simulink model "sst_three_phase_dab_three_levels_inv"  (R2025b)
settings: Solver=ode23tb  StartTime=0.0  StopTime=simlength  FixedStep=tc  MaxStep=tc
values from neighbouring files (symbols this model uses):
  Adrso = eye(2) + Arso*ts_inv    [init_model.m]
  Aresd_max = eye(2) + Ares_max*ts_afe    [init_model.m]
  Aresd_min = eye(2) + Ares_min*ts_afe    [init_model.m]
  Aresd_nom = eye(2) + Ares_nom*ts_afe    [init_model.m]
  Bresd = Bres*ts_afe    [init_model.m]
  CFi_dc2 = 900e-6*4    (= 0.0036)    [init_model.m]
  Cresd = Cres    [init_model.m]
  Crso = [1 0]    [init_model.m]
  delta = 0.025    [init_model.m]
  freq = 50    [init_model.m]
  Iac_FS = I_phase_normalization_factor    [init_model.m]
  Idc_FS = max(Idab1_dc_nom,Idab2_dc_nom) * margin_factor    [init_model.m]
  iph_grid_pu_ref = 3.75    [init_model.m]
  ki_afe = 18    [init_model.m]
  ki_pll = 3140    [init_model.m]
  ki_rpi = 18    [init_model.m]
  kp_afe = 0.25    [init_model.m]
  kp_pll = 314    [init_model.m]
  kp_rpi = 0.25    [init_model.m]
  Ldrso = acker(Adrso',Crso',polesdrso)'    [init_model.m]
  LFu1_AFE = 0.33e-3    (= 0.00033)    [init_model.m]
  n_modules = 2    [init_model.m]
  RLFu1_AFE = 157*0.05*LFu1_AFE    (= 0.0025905)    [init_model.m]
  tc = ts_dab/1000*24    (= 1e-06)    [init_model.m]
  ts_afe = 1/fPWM_AFE    (= 0.00025)    [init_model.m]
  ts_inv = 1/fPWM_INV    (= 0.00025)    [init_model.m]
  Vac_FS = V_phase_normalization_factor    [init_model.m]
  Vdab2_dc_nom = 1500    [init_model.m]
  Vdc_FS = max(Vdab1_dc_nom,Vdab2_dc_nom) * margin_factor    [init_model.m]
undefined symbols (not defined in the file or in its folder): omega_grid_nom, V_phase_normalization_factor
libraries: fl_lib x80, nesl_utility x55, discrete_time_low_pass_filter x6, single_phase_transformer x6, pi_ctrl x4, three_phase_inverter_ideal_switch_based_model x4, three_phase_inverter_mosfet_based_with_thermal_model x4, single_phase_transformer_lib x3, three_phase_dab_modulator x2, dclink_for_three_levels x2, single_phase_three_levels_PWM_modulator x2, dq_vector_pi x2
(part 3 of 5)

== system sst_three_phase_dab_three_levels_inv/inverter_modB/single phase inverter control1/acquisition_and_scaling_current ==
  in : Inport
  1/Ti5 : Gain  Gain=1/Iac_FS  SaturateOnIntegerOverflow=on  OutDataTypeStr=Inherit: Same as input  ParamDataTypeStr=Inherit: Same as input
  out : Outport
  wires:
  in/1 -> 1/Ti5/1
  1/Ti5/1 -> out/1

== system sst_three_phase_dab_three_levels_inv/inverter_modB/single phase inverter control1/acquisition_and_scaling_dc_voltage ==
  in : Inport
  1/Ti3 : Gain  Gain=1/Vdc_FS  SaturateOnIntegerOverflow=on  OutDataTypeStr=Inherit: Same as input  ParamDataTypeStr=Inherit: Same as input
  out : Outport
  wires:
  in/1 -> 1/Ti3/1
  1/Ti3/1 -> out/1

== system sst_three_phase_dab_three_levels_inv/inverter_modB/single phase inverter control1/acquisition_and_scaling_voltage ==
  in : Inport
  1/Ti5 : Gain  Gain=1/Vac_FS  SaturateOnIntegerOverflow=on  OutDataTypeStr=Inherit: Same as input  ParamDataTypeStr=Inherit: Same as input
  out : Outport
  wires:
  in/1 -> 1/Ti5/1
  1/Ti5/1 -> out/1

== system sst_three_phase_dab_three_levels_inv/inverter_modB/single phase inverter control1/acquisition_and_scaling_voltage1 ==
  in : Inport
  1/Ti1 : Gain  Gain=1/Vac_FS  SaturateOnIntegerOverflow=on  OutDataTypeStr=Inherit: Same as input  ParamDataTypeStr=Inherit: Same as input
  1/Ti2 : Gain  Gain=1/n_modules  SaturateOnIntegerOverflow=on  OutDataTypeStr=Inherit: Same as input  ParamDataTypeStr=Inherit: Same as input
  out : Outport
  wires:
  in/1 -> 1/Ti2/1
  1/Ti1/1 -> out/1
  1/Ti2/1 -> 1/Ti1/1

== system sst_three_phase_dab_three_levels_inv/inverter_modB/single phase inverter control1/inverter_current_output_pu_reference ==
  Gain : Gain
  Rate Limiter : RateLimiter  RisingSlewLimit=50  FallingSlewLimit=-50  SampleTimeMode=inherited
  Sum : Sum  Inputs=|++
  i_out_inverter_reference_step1 : Step  Time=0.05  After=iph_grid_pu_ref  SampleTime=0
  i_out_inverter_reference_step2 : Step  Commented=on  Time=0.25  After=-iph_grid_pu_ref  SampleTime=0
  inverter_current_output_pu_reference : Outport
  wires:
  Rate Limiter/1 -> Gain/1
  Sum/1 -> Rate Limiter/1
  i_out_inverter_reference_step1/1 -> Sum/1
  i_out_inverter_reference_step2/1 -> Sum/2
  Gain/1 -> inverter_current_output_pu_reference/1

== system sst_three_phase_dab_three_levels_inv/inverter_modB/single phase inverter control1/pwm modulator ==
  vout : Inport
  Constant : Constant  Value=0
  single_phase_three_levels_PWM_generator_with_global_TRGO : single_phase_three_levels_PWM_modulator/single_phase_three_levels_PWM_generator_with_global_TRGO  f=fPWM_INV  m_up=1  m_low=-1  dead_time=dead_time_INV  pos_cmd_gate=15  neg_cmd_gate=-10  polarity=1  tc=tc  double_sampling=1
  gate_cmds : Outport
  tag scope: TRGO_INV_2=global
  wires:
  vout/1 -> single_phase_three_levels_PWM_generator_with_global_TRGO/3
  Constant/1 -> single_phase_three_levels_PWM_generator_with_global_TRGO/2
  single_phase_three_levels_PWM_generator_with_global_TRGO/2 -> gate_cmds/1
  single_phase_three_levels_PWM_generator_with_global_TRGO/1 -> [TRGO_INV_2]
  [time_afe_module_2] -> single_phase_three_levels_PWM_generator_with_global_TRGO/1

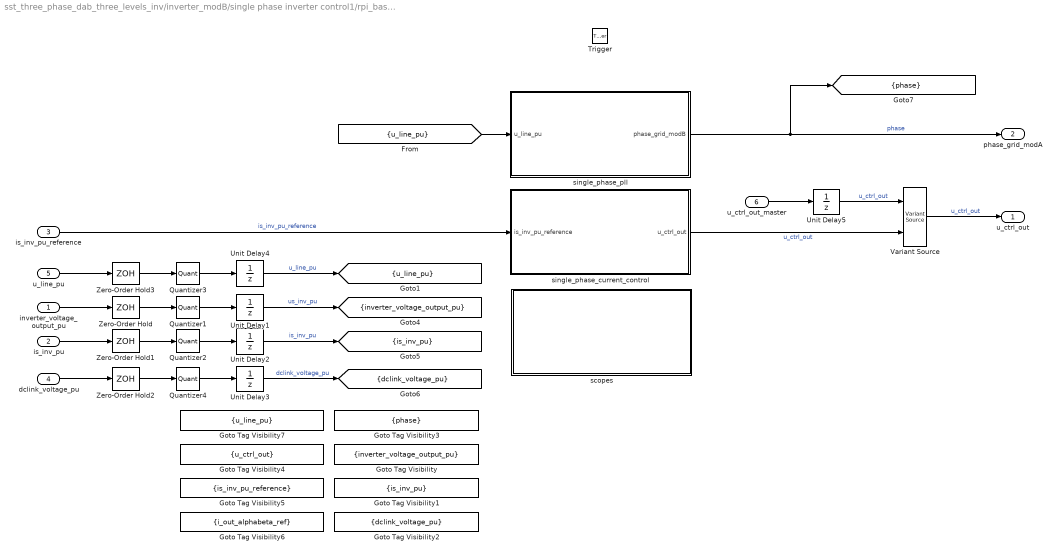
== system sst_three_phase_dab_three_levels_inv/inverter_modB/single phase inverter control1/rpi_based_single_phase_inverter_ctrl ==
  inverter_voltage_output_pu : Inport
  is_inv_pu : Inport  Port=2
  is_inv_pu_reference : Inport  Port=3
  dclink_voltage_pu : Inport  Port=4
  u_line_pu : Inport  Port=5
  u_ctrl_out_master : Inport  Port=6
  Trigger : TriggerPort  VariantControl=(inherit)  PortDimensions=1
  Goto Tag Visibility : GotoTagVisibility  GotoTag=inverter_voltage_output_pu
  Goto Tag Visibility1 : GotoTagVisibility  GotoTag=is_inv_pu
  Goto Tag Visibility2 : GotoTagVisibility  GotoTag=dclink_voltage_pu
  Goto Tag Visibility3 : GotoTagVisibility  GotoTag=phase
  Goto Tag Visibility4 : GotoTagVisibility  GotoTag=u_ctrl_out
  Goto Tag Visibility5 : GotoTagVisibility  GotoTag=is_inv_pu_reference
  Goto Tag Visibility6 : GotoTagVisibility  GotoTag=i_out_alphabeta_ref
  Goto Tag Visibility7 : GotoTagVisibility  GotoTag=u_line_pu
  Quantizer{1..4} (4 alike) : Quantizer  QuantizationInterval=adc12_quantization
  Unit Delay{1..5} (5 alike) : UnitDelay  SampleTime=-1  HasFrameUpgradeWarning=on
  Variant Source : VariantSource  VariantControls={true, false}
  Zero-Order Hold{,1..3} (4 alike) : ZeroOrderHold  SampleTime=-1
  scopes : Subsystem
  single_phase_current_control : Subsystem
  single_phase_pll : Subsystem
  u_ctrl_out : Outport
  phase_grid_modA : Outport  Port=2
  tag scope: dclink_voltage_pu=scoped, inverter_voltage_output_pu=scoped, is_inv_pu=scoped, phase=scoped, u_line_pu=scoped
  wires:
  inverter_voltage_output_pu/1 -> Zero-Order Hold/1
  is_inv_pu/1 -> Zero-Order Hold1/1
  dclink_voltage_pu/1 -> Zero-Order Hold2/1
  Unit Delay1/1 -> [inverter_voltage_output_pu]  "us_inv_pu"
  Unit Delay2/1 -> [is_inv_pu]  "is_inv_pu"
  Unit Delay3/1 -> [dclink_voltage_pu]  "dclink_voltage_pu"
  is_inv_pu_reference/1 -> single_phase_current_control/1(is_inv_pu_reference)  "is_inv_pu_reference"
  u_line_pu/1 -> Zero-Order Hold3/1
  Quantizer1/1 -> Unit Delay1/1
  Quantizer2/1 -> Unit Delay2/1
  Quantizer4/1 -> Unit Delay3/1
  Quantizer3/1 -> Unit Delay4/1
  single_phase_pll/1(phase_grid_modB) -> [phase], phase_grid_modA/1  "phase"
  Zero-Order Hold/1 -> Quantizer1/1
  Zero-Order Hold1/1 -> Quantizer2/1
  Zero-Order Hold2/1 -> Quantizer4/1
  Unit Delay4/1 -> [u_line_pu]  "u_line_pu"
  [u_line_pu] -> single_phase_pll/1(u_line_pu)
  Zero-Order Hold3/1 -> Quantizer3/1
  u_ctrl_out_master/1 -> Unit Delay5/1
  Unit Delay5/1 -> Variant Source/1  "u_ctrl_out"
  Variant Source/1 -> u_ctrl_out/1  "u_ctrl_out"
  single_phase_current_control/1(u_ctrl_out) -> Variant Source/2  "u_ctrl_out"

== system sst_three_phase_dab_three_levels_inv/dab_modA/dab_ctrl/ui_ctrl/dab_ctrl ==
  i_pu_dab_input : Inport
  u_pu_dab_output : Inport  Port=2
  u_pu_dab_output_ref : Inport  Port=3
  Quantizer1 : Quantizer  QuantizationInterval=adc12_quantization
  Quantizer2 : Quantizer  QuantizationInterval=adc12_quantization
  Unit Delay1 : UnitDelay  SampleTime=-1  HasFrameUpgradeWarning=on
  Unit Delay2 : UnitDelay  SampleTime=-1  HasFrameUpgradeWarning=on
  Unit Delay3 : UnitDelay  SampleTime=-1  HasFrameUpgradeWarning=on
  Vout Ctrl : Subsystem
  current control : Subsystem
  discrete-time-low-pass-filter6 : discrete_time_low_pass_filter/discrete-time-low-pass-filter  tau=0.02  ts=ts_dab
  phase_displacement : Outport
  tag scope: i_ctrl_out_dab=scoped, i_in_pu_dab=scoped, u_ctrl_out_dab=scoped, uout_pu_dab=scoped, uout_ref_pu_dab=scoped
  wires:
  Vout Ctrl/1(ctrlv_out) -> [u_ctrl_out_dab], current control/1(iout_ref)  "iout_ref"
  i_pu_dab_input/1 -> Quantizer2/1
  current control/1(i_ctrl_out) -> phase_displacement/1, [i_ctrl_out_dab]
  Unit Delay3/1 -> current control/2(iout), [i_in_pu_dab]
  Unit Delay2/1 -> [uout_pu_dab], Vout Ctrl/2(vout)
  Unit Delay1/1 -> Vout Ctrl/1(vout_ref), [uout_ref_pu_dab]
  u_pu_dab_output/1 -> Quantizer1/1
  u_pu_dab_output_ref/1 -> discrete-time-low-pass-filter6/1
  Quantizer1/1 -> Unit Delay2/1
  Quantizer2/1 -> Unit Delay3/1
  discrete-time-low-pass-filter6/1 -> Unit Delay1/1

== system sst_three_phase_dab_three_levels_inv/dab_modA/dab_ctrl/ui_ctrl/scopes ==
  Bus Creator : BusCreator  Inputs=2
  Bus Creator1 : BusCreator  Inputs=2
  dab-tracking : Scope  NumInputPorts=2
      settings: ActiveDisplayYMinimum=-1.24267578125  ActiveDisplayYMaximum=0.54443359375  DataLoggingVariableName=ScopeData7
  u_ctrl_out_dab/i_ctrl_out_dab : Scope  NumInputPorts=2
      settings: ActiveDisplayYMinimum=-1.2812486231311795  ActiveDisplayYMaximum=1.531237608180616
  wires:
  Bus Creator1/1 -> dab-tracking/2
  Bus Creator/1 -> dab-tracking/1
  [i_ctrl_out_dab] -> u_ctrl_out_dab/i_ctrl_out_dab/2  "i_ctrl_out_dab"
  [i_in_pu_dab] -> Bus Creator1/2  "i_in_pu_dab"
  [uout_ref_pu_dab] -> Bus Creator/1  "uout_ref_pu_dab"
  [u_ctrl_out_dab] -> u_ctrl_out_dab/i_ctrl_out_dab/1  "u_ctrl_out_dab"
  [u_ctrl_out_dab] -> Bus Creator1/1  "u_ctrl_out_dab"
  [uout_pu_dab] -> Bus Creator/2  "uout_pu_dab"

== system sst_three_phase_dab_three_levels_inv/dab_modA/dab_ctrl/ui_ctrl/storage_data ==
  To Workspace1 : ToWorkspace  VariableName=time_ts_dab_modA_sim  SampleTime=-1
      settings: MaxDataPoints=Ns_dab
  To Workspace2 : ToWorkspace  VariableName=i_in_pu_dab_modA_sim  SampleTime=-1
      settings: MaxDataPoints=Ns_dab
  To Workspace3 : ToWorkspace  VariableName=i_in_pu_ref_dab_modA_sim  SampleTime=-1
      settings: MaxDataPoints=Ns_dab
  To Workspace4 : ToWorkspace  VariableName=i_ctrl_out_dab_modA_sim  SampleTime=-1
      settings: MaxDataPoints=Ns_dab
  wires:
  [u_ctrl_out_dab] -> To Workspace3/1  "u_ctrl_out_dab"
  [i_ctrl_out_dab] -> To Workspace4/1  "i_ctrl_out_dab"
  [i_in_pu_dab] -> To Workspace2/1  "i_in_pu_dab"
  [local_time] -> To Workspace1/1  "local_time"

== system sst_three_phase_dab_three_levels_inv/dab_modA/dcdc_with_galvanic_isolation/single_phase_dab_transformer/three_phase_hf_transformer ==
  single_phase_transformer_1 : single_phase_transformer/single_phase_transformer  lm_trafo=lm_trafo  m1=m1  m2=m2  rd1_trafo=rd1_trafo  rd2_trafo=rd2_trafo  ld1_trafo=ld1_trafo  ld2_trafo=ld2_trafo  rfe_trafo=rfe_trafo  length_core=1  mu0=1.256637e-6  mur=10e3
  single_phase_transformer_2 : single_phase_transformer/single_phase_transformer  lm_trafo=lm_trafo  m1=m1  m2=m2  rd1_trafo=rd1_trafo  rd2_trafo=rd2_trafo  ld1_trafo=ld1_trafo  ld2_trafo=ld2_trafo  rfe_trafo=rfe_trafo  length_core=1  mu0=1.256637e-6  mur=10e3
  single_phase_transformer_2: data : Scope
      settings: ActiveDisplayYMinimum=-1744.0416508829171  ActiveDisplayYMaximum=1756.9104494327478  DataLoggingVariableName=ScopeData15
  single_phase_transformer_3 : single_phase_transformer/single_phase_transformer  lm_trafo=lm_trafo  m1=m1  m2=m2  rd1_trafo=rd1_trafo  rd2_trafo=rd2_trafo  ld1_trafo=ld1_trafo  ld2_trafo=ld2_trafo  rfe_trafo=rfe_trafo  length_core=1  mu0=1.256637e-6  mur=10e3
  ua1 : PMIOPort  Side=Left
  ua2 : PMIOPort  Port=2  Side=Right
  ub1 : PMIOPort  Port=3  Side=Left
  ub2 : PMIOPort  Port=4  Side=Right
  uc1 : PMIOPort  Port=5  Side=Left
  uc2 : PMIOPort  Port=6  Side=Right
  un1 : PMIOPort  Port=7  Side=Left
  un2 : PMIOPort  Port=8  Side=Right
  wires:
  single_phase_transformer_2/1 -> single_phase_transformer_2: data/1
  connections:
  un2/RConn1 -- single_phase_transformer_2/RConn2 -- single_phase_transformer_1/RConn2 -- single_phase_transformer_3/RConn2
  un1/RConn1 -- single_phase_transformer_2/LConn2 -- single_phase_transformer_1/LConn2 -- single_phase_transformer_3/LConn2
  single_phase_transformer_1/LConn1 -- ua1/RConn1
  single_phase_transformer_2/LConn1 -- ub1/RConn1
  single_phase_transformer_3/LConn1 -- uc1/RConn1
  single_phase_transformer_3/RConn1 -- uc2/RConn1
  single_phase_transformer_2/RConn1 -- ub2/RConn1
  single_phase_transformer_1/RConn1 -- ua2/RConn1

== system sst_three_phase_dab_three_levels_inv/dab_modA/dcdc_with_galvanic_isolation/single_phase_dab_transformer/three_phase_hf_transformer1 ==
  tr1 : single_phase_transformer_lib/single phase transformer  Lm=lm_trafo H  n1=m1  n2=m2  Rd1=rd1_trafo Ohm  Rd2=rd2_trafo Ohm  Ld1=ld1_trafo H  Ld2=ld2_trafo H  Rfe=rfe_trafo Ohm  phi_specify=off  phi_priority=None  phi=0 V*s  phi_nominal_specify=off  phi_nominal_value=1  phi_nominal_unit=V*s  i1_specify=on  i1_priority=High  i1=0 A  i1_nominal_specify=off  i1_nominal_value=1  i1_nominal_unit=A  i2_specify=on  i2_priority=High  i2=0 A  i2_nominal_specify=off  i2_nominal_value=1  i2_nominal_unit=A  ife_specify=off  ife_priority=None  ife=0 A  ife_nominal_specify=off  ife_nominal_value=1  ife_nominal_unit=A  u1_specify=off  u1_priority=None  u1=0 V  u1_nominal_specify=off  u1_nominal_value=1  u1_nominal_unit=V  u2_specify=off  u2_priority=None  u2=0 V  u2_nominal_specify=off  u2_nominal_value=1  u2_nominal_unit=V
      settings: InternalSimscapePortConfiguration="{\"Bottom\":[],\"Left\":[{\"id\":\"u1_p\",\"label\":\"u1(+)\",\"type\":\"foundation.electrical.electrical\"},{\"id\":\"u1_n\",\"label\":\"u1(-)\",\"type\":\"foundation.electrical.electrical\"}],\"Right\":[{\"id\":\"u2_p\",\"label\":\"u2(+)\",\"type\":\"foundation.electrical.electrical\"},{\"id\":\"u2_n\",\"label\":\"u2(-)\",\"type\":\"foundation.electrical.electrical\"}],\"Top\":[]}"
  tr2 : single_phase_transformer_lib/single phase transformer  Lm=lm_trafo H  n1=m1  n2=m2  Rd1=rd1_trafo Ohm  Rd2=rd2_trafo Ohm  Ld1=ld1_trafo H  Ld2=ld2_trafo H  Rfe=rfe_trafo Ohm  phi_specify=off  phi_priority=None  phi=0 V*s  phi_nominal_specify=off  phi_nominal_value=1  phi_nominal_unit=V*s  i1_specify=on  i1_priority=High  i1=0 A  i1_nominal_specify=off  i1_nominal_value=1  i1_nominal_unit=A  i2_specify=on  i2_priority=High  i2=0 A  i2_nominal_specify=off  i2_nominal_value=1  i2_nominal_unit=A  ife_specify=off  ife_priority=None  ife=0 A  ife_nominal_specify=off  ife_nominal_value=1  ife_nominal_unit=A  u1_specify=off  u1_priority=None  u1=0 V  u1_nominal_specify=off  u1_nominal_value=1  u1_nominal_unit=V  u2_specify=off  u2_priority=None  u2=0 V  u2_nominal_specify=off  u2_nominal_value=1  u2_nominal_unit=V
      settings: InternalSimscapePortConfiguration="{\"Bottom\":[],\"Left\":[{\"id\":\"u1_p\",\"label\":\"u1(+)\",\"type\":\"foundation.electrical.electrical\"},{\"id\":\"u1_n\",\"label\":\"u1(-)\",\"type\":\"foundation.electrical.electrical\"}],\"Right\":[{\"id\":\"u2_p\",\"label\":\"u2(+)\",\"type\":\"foundation.electrical.electrical\"},{\"id\":\"u2_n\",\"label\":\"u2(-)\",\"type\":\"foundation.electrical.electrical\"}],\"Top\":[]}"
  tr3 : single_phase_transformer_lib/single phase transformer  Lm=lm_trafo H  n1=m1  n2=m2  Rd1=rd1_trafo Ohm  Rd2=rd2_trafo Ohm  Ld1=ld1_trafo H  Ld2=ld2_trafo H  Rfe=rfe_trafo Ohm  phi_specify=off  phi_priority=None  phi=0 V*s  phi_nominal_specify=off  phi_nominal_value=1  phi_nominal_unit=V*s  i1_specify=on  i1_priority=High  i1=0 A  i1_nominal_specify=off  i1_nominal_value=1  i1_nominal_unit=A  i2_specify=on  i2_priority=High  i2=0 A  i2_nominal_specify=off  i2_nominal_value=1  i2_nominal_unit=A  ife_specify=off  ife_priority=None  ife=0 A  ife_nominal_specify=off  ife_nominal_value=1  ife_nominal_unit=A  u1_specify=off  u1_priority=None  u1=0 V  u1_nominal_specify=off  u1_nominal_value=1  u1_nominal_unit=V  u2_specify=off  u2_priority=None  u2=0 V  u2_nominal_specify=off  u2_nominal_value=1  u2_nominal_unit=V
      settings: InternalSimscapePortConfiguration="{\"Bottom\":[],\"Left\":[{\"id\":\"u1_p\",\"label\":\"u1(+)\",\"type\":\"foundation.electrical.electrical\"},{\"id\":\"u1_n\",\"label\":\"u1(-)\",\"type\":\"foundation.electrical.electrical\"}],\"Right\":[{\"id\":\"u2_p\",\"label\":\"u2(+)\",\"type\":\"foundation.electrical.electrical\"},{\"id\":\"u2_n\",\"label\":\"u2(-)\",\"type\":\"foundation.electrical.electrical\"}],\"Top\":[]}"
  ua1 : PMIOPort  Side=Left
  ua2 : PMIOPort  Port=2  Side=Right
  ub1 : PMIOPort  Port=3  Side=Left
  ub2 : PMIOPort  Port=4  Side=Right
  uc1 : PMIOPort  Port=5  Side=Left
  uc2 : PMIOPort  Port=6  Side=Right
  un1 : PMIOPort  Port=7  Side=Left
  un2 : PMIOPort  Port=8  Side=Right
  connections:
  uc2/RConn1 -- tr3/RConn1
  uc1/RConn1 -- tr3/LConn1
  ua1/RConn1 -- tr1/LConn1
  tr1/RConn1 -- ua2/RConn1
  ub2/RConn1 -- tr2/RConn1
  un1/RConn1 -- tr3/LConn2 -- tr2/LConn2 -- tr1/LConn2
  un2/RConn1 -- tr3/RConn2 -- tr2/RConn2 -- tr1/RConn2
  ub1/RConn1 -- tr2/LConn1

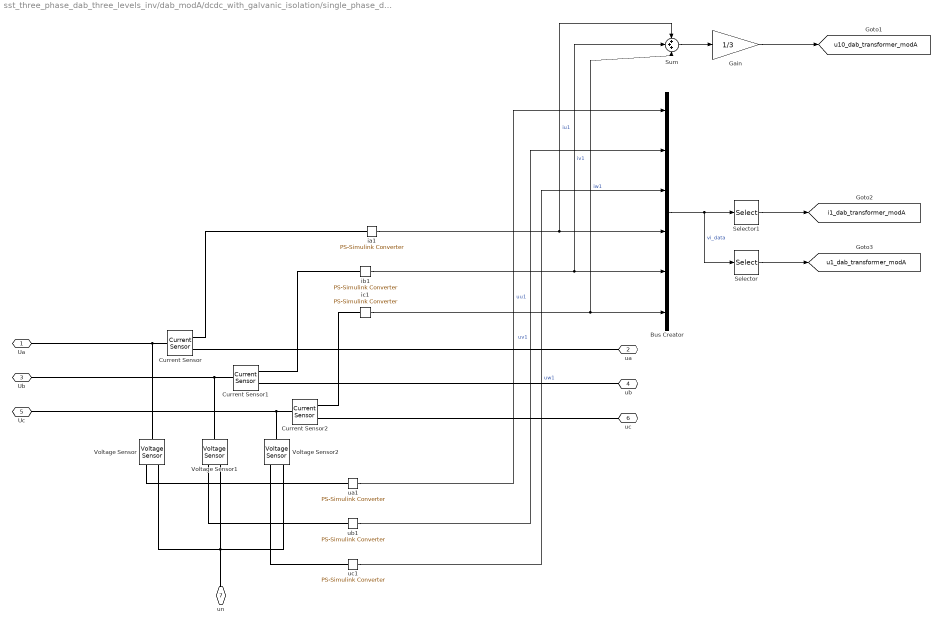
== system sst_three_phase_dab_three_levels_inv/dab_modA/dcdc_with_galvanic_isolation/single_phase_dab_transformer/threephase_vi_measures_stack ==
  Bus Creator : BusCreator  Inputs=6
  Current Sensor : fl_lib/Electrical/Electrical Sensors/Current Sensor
  Current Sensor1 : fl_lib/Electrical/Electrical Sensors/Current Sensor
  Current Sensor2 : fl_lib/Electrical/Electrical Sensors/Current Sensor
  Gain : Gain  Gain=1/3
  Selector : Selector  InputPortWidth=6  IndexOptions=Index vector (dialog)  Indices=[1 2 3]  OutputSizes=1
  Selector1 : Selector  InputPortWidth=6  IndexOptions=Index vector (dialog)  Indices=[4 5 6]  OutputSizes=1
  Sum : Sum  Inputs=+++
  Voltage Sensor : fl_lib/Electrical/Electrical Sensors/Voltage Sensor
  Voltage Sensor1 : fl_lib/Electrical/Electrical Sensors/Voltage Sensor
  Voltage Sensor2 : fl_lib/Electrical/Electrical Sensors/Voltage Sensor
  ia1 : nesl_utility/PS-Simulink Converter  PhysicalDomain=network_engine_domain  SubClassName=ps_output  LeftPortType=input  RightPortType=output  PseudoPeriodic=off  Frequencies=[]  VectorFormat=1-D array  Unit=A  AffineConversion=off
  ib1 : nesl_utility/PS-Simulink Converter  PhysicalDomain=network_engine_domain  SubClassName=ps_output  LeftPortType=input  RightPortType=output  PseudoPeriodic=off  Frequencies=[]  VectorFormat=1-D array  Unit=A  AffineConversion=off
  ic1 : nesl_utility/PS-Simulink Converter  PhysicalDomain=network_engine_domain  SubClassName=ps_output  LeftPortType=input  RightPortType=output  PseudoPeriodic=off  Frequencies=[]  VectorFormat=1-D array  Unit=A  AffineConversion=off
  ua1 : nesl_utility/PS-Simulink Converter  PhysicalDomain=network_engine_domain  SubClassName=ps_output  LeftPortType=input  RightPortType=output  PseudoPeriodic=off  Frequencies=[]  VectorFormat=1-D array  Unit=V  AffineConversion=off
  ub1 : nesl_utility/PS-Simulink Converter  PhysicalDomain=network_engine_domain  SubClassName=ps_output  LeftPortType=input  RightPortType=output  PseudoPeriodic=off  Frequencies=[]  VectorFormat=1-D array  Unit=V  AffineConversion=off
  uc1 : nesl_utility/PS-Simulink Converter  PhysicalDomain=network_engine_domain  SubClassName=ps_output  LeftPortType=input  RightPortType=output  PseudoPeriodic=off  Frequencies=[]  VectorFormat=1-D array  Unit=V  AffineConversion=off
  Ua : PMIOPort  Side=Left
  ua : PMIOPort  Port=2  Side=Right
  Ub : PMIOPort  Port=3  Side=Left
  ub : PMIOPort  Port=4  Side=Right
  Uc : PMIOPort  Port=5  Side=Left
  uc : PMIOPort  Port=6  Side=Right
  un : PMIOPort  Port=7  Side=Right
  tag scope: i1_dab_transformer_modA=global, u10_dab_transformer_modA=global, u1_dab_transformer_modA=global
  wires:
  Bus Creator/1 -> Selector/1, Selector1/1  "vi_data"
  Selector/1 -> [u1_dab_transformer_modA]
  ib1/1 -> Sum/2, Bus Creator/5  "iv1"
  ia1/1 -> Sum/1, Bus Creator/4  "iu1"
  ic1/1 -> Bus Creator/6, Sum/3  "iw1"
  ua1/1 -> Bus Creator/1  "uu1"
  ub1/1 -> Bus Creator/2  "uv1"
  uc1/1 -> Bus Creator/3  "uw1"
  Selector1/1 -> [i1_dab_transformer_modA]
  Sum/1 -> Gain/1
  Gain/1 -> [u10_dab_transformer_modA]
  connections:
  Current Sensor1/LConn1 -- Ub/RConn1 -- Voltage Sensor1/LConn1
  Voltage Sensor/RConn2 -- un/RConn1 -- Voltage Sensor2/RConn2 -- Voltage Sensor1/RConn2
  Voltage Sensor/RConn1 -- ua1/LConn1
  Current Sensor/RConn2 -- ua/RConn1
  Voltage Sensor1/RConn1 -- ub1/LConn1
  Voltage Sensor2/LConn1 -- Uc/RConn1 -- Current Sensor2/LConn1
  Current Sensor/LConn1 -- Ua/RConn1 -- Voltage Sensor/LConn1
  Current Sensor1/RConn2 -- ub/RConn1
  Voltage Sensor2/RConn1 -- uc1/LConn1
  ib1/LConn1 -- Current Sensor1/RConn1
  ia1/LConn1 -- Current Sensor/RConn1
  ic1/LConn1 -- Current Sensor2/RConn1
  Current Sensor2/RConn2 -- uc/RConn1

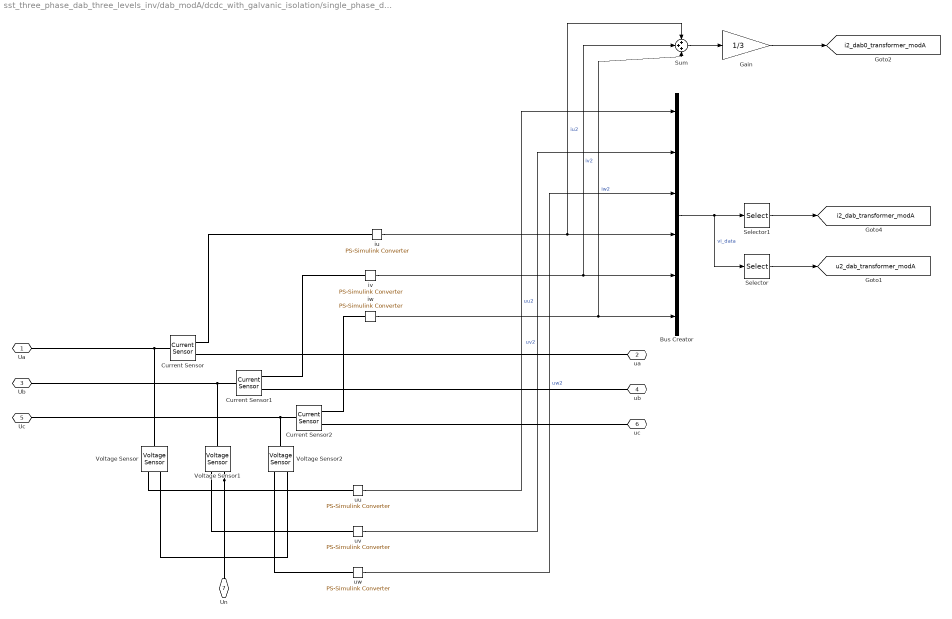
== system sst_three_phase_dab_three_levels_inv/dab_modA/dcdc_with_galvanic_isolation/single_phase_dab_transformer/threephase_vi_measures_stack1 ==
  Bus Creator : BusCreator  Inputs=6
  Current Sensor : fl_lib/Electrical/Electrical Sensors/Current Sensor
  Current Sensor1 : fl_lib/Electrical/Electrical Sensors/Current Sensor
  Current Sensor2 : fl_lib/Electrical/Electrical Sensors/Current Sensor
  Gain : Gain  Gain=1/3
  Selector : Selector  InputPortWidth=6  IndexOptions=Index vector (dialog)  Indices=[1 2 3]  OutputSizes=1
  Selector1 : Selector  InputPortWidth=6  IndexOptions=Index vector (dialog)  Indices=[4 5 6]  OutputSizes=1
  Sum : Sum  Inputs=+++
  Voltage Sensor : fl_lib/Electrical/Electrical Sensors/Voltage Sensor
  Voltage Sensor1 : fl_lib/Electrical/Electrical Sensors/Voltage Sensor
  Voltage Sensor2 : fl_lib/Electrical/Electrical Sensors/Voltage Sensor
  iu : nesl_utility/PS-Simulink Converter  PhysicalDomain=network_engine_domain  SubClassName=ps_output  LeftPortType=input  RightPortType=output  PseudoPeriodic=off  Frequencies=[]  VectorFormat=1-D array  Unit=A  AffineConversion=off
  iv : nesl_utility/PS-Simulink Converter  PhysicalDomain=network_engine_domain  SubClassName=ps_output  LeftPortType=input  RightPortType=output  PseudoPeriodic=off  Frequencies=[]  VectorFormat=1-D array  Unit=A  AffineConversion=off
  iw : nesl_utility/PS-Simulink Converter  PhysicalDomain=network_engine_domain  SubClassName=ps_output  LeftPortType=input  RightPortType=output  PseudoPeriodic=off  Frequencies=[]  VectorFormat=1-D array  Unit=A  AffineConversion=off
  uu : nesl_utility/PS-Simulink Converter  PhysicalDomain=network_engine_domain  SubClassName=ps_output  LeftPortType=input  RightPortType=output  PseudoPeriodic=off  Frequencies=[]  VectorFormat=1-D array  Unit=V  AffineConversion=off
  uv : nesl_utility/PS-Simulink Converter  PhysicalDomain=network_engine_domain  SubClassName=ps_output  LeftPortType=input  RightPortType=output  PseudoPeriodic=off  Frequencies=[]  VectorFormat=1-D array  Unit=V  AffineConversion=off
  uw : nesl_utility/PS-Simulink Converter  PhysicalDomain=network_engine_domain  SubClassName=ps_output  LeftPortType=input  RightPortType=output  PseudoPeriodic=off  Frequencies=[]  VectorFormat=1-D array  Unit=V  AffineConversion=off
  Ua : PMIOPort  Side=Left
  ua : PMIOPort  Port=2  Side=Right
  Ub : PMIOPort  Port=3  Side=Left
  ub : PMIOPort  Port=4  Side=Right
  Uc : PMIOPort  Port=5  Side=Left
  uc : PMIOPort  Port=6  Side=Right
  Un : PMIOPort  Port=7  Side=Left
  tag scope: i2_dab0_transformer_modA=global, i2_dab_transformer_modA=global, u2_dab_transformer_modA=global
  wires:
  uu/1 -> Bus Creator/1  "uu2"
  Gain/1 -> [i2_dab0_transformer_modA]
  Sum/1 -> Gain/1
  Selector1/1 -> [i2_dab_transformer_modA]
  uw/1 -> Bus Creator/3  "uw2"
  uv/1 -> Bus Creator/2  "uv2"
  iw/1 -> Bus Creator/6, Sum/3  "iw2"
  iu/1 -> Bus Creator/4, Sum/1  "iu2"
  iv/1 -> Bus Creator/5, Sum/2  "iv2"
  Selector/1 -> [u2_dab_transformer_modA]
  Bus Creator/1 -> Selector1/1, Selector/1  "vi_data"
  connections:
  Current Sensor2/RConn2 -- uc/RConn1
  iw/LConn1 -- Current Sensor2/RConn1
  iu/LConn1 -- Current Sensor/RConn1
  iv/LConn1 -- Current Sensor1/RConn1
  Voltage Sensor2/RConn1 -- uw/LConn1
  Current Sensor1/RConn2 -- ub/RConn1
  Voltage Sensor/LConn1 -- Ua/RConn1 -- Current Sensor/LConn1
  Current Sensor2/LConn1 -- Uc/RConn1 -- Voltage Sensor2/LConn1
  Voltage Sensor1/RConn1 -- uv/LConn1
  Current Sensor/RConn2 -- ua/RConn1
  Voltage Sensor/RConn1 -- uu/LConn1
  Voltage Sensor1/RConn2 -- Un/RConn1 -- Voltage Sensor2/RConn2 -- Voltage Sensor/RConn2
  Voltage Sensor1/LConn1 -- Ub/RConn1 -- Current Sensor1/LConn1

== system sst_three_phase_dab_three_levels_inv/dab_modA/dcdc_with_galvanic_isolation/three_phase_inverter_1/dclink_1 ==
  CFi_dc1 : fl_lib/Electrical/Electrical Elements/Capacitor  c=CFi_dc1 F  r=RCFi_dc1_internal Ohm  g=0 1/Ohm  i_specify=off  i_priority=None  i=0 A  i_nominal_specify=off  i_nominal_value=1  i_nominal_unit=A  v_specify=off  v_priority=None  v=0 V  v_nominal_specify=off  v_nominal_value=1  v_nominal_unit=V  vc_specify=off  vc_priority=High  vc=0 V  vc_nominal_specify=off  vc_nominal_value=1  vc_nominal_unit=V
  Current Sensor : fl_lib/Electrical/Electrical Sensors/Current Sensor
  PS-Simulink Converter1 : nesl_utility/PS-Simulink Converter  PhysicalDomain=network_engine_domain  SubClassName=ps_output  LeftPortType=input  RightPortType=output  PseudoPeriodic=off  Frequencies=[]  VectorFormat=1-D array  Unit=A  AffineConversion=on
  PS-Simulink Converter4 : nesl_utility/PS-Simulink Converter  PhysicalDomain=network_engine_domain  SubClassName=ps_output  LeftPortType=input  RightPortType=output  PseudoPeriodic=off  Frequencies=[]  VectorFormat=1-D array  Unit=V  AffineConversion=on
  Voltage Sensor : fl_lib/Electrical/Electrical Sensors/Voltage Sensor
  udc(+) : PMIOPort  Side=Left
  Udc(+) : PMIOPort  Port=2  Side=Right
  udc(-) : PMIOPort  Port=3  Side=Left
  Udc(-) : PMIOPort  Port=4  Side=Right
  tag scope: CFi_dc1_current_modA=global, dab_voltage_input_modA=global
  wires:
  PS-Simulink Converter4/1 -> [dab_voltage_input_modA]  "dab_voltage_input_modA"
  PS-Simulink Converter1/1 -> [CFi_dc1_current_modA]  "CFi_dc_current"
  connections:
  Current Sensor/RConn1 -- PS-Simulink Converter1/LConn1
  PS-Simulink Converter4/LConn1 -- Voltage Sensor/RConn1
  Current Sensor/LConn1 -- CFi_dc1/RConn1
  Voltage Sensor/RConn2 -- Current Sensor/RConn2 -- Udc(-)/RConn1 -- udc(-)/RConn1
  CFi_dc1/LConn1 -- Udc(+)/RConn1 -- udc(+)/RConn1 -- Voltage Sensor/LConn1

== system sst_three_phase_dab_three_levels_inv/dab_modA/dcdc_with_galvanic_isolation/three_phase_inverter_1/three_phase_inverter_1 ==
  gate_commands : Inport
  three_phase_inverter_ideal_switch_based_model : three_phase_inverter_ideal_switch_based_model/three phase inverter ideal switch based model  Commented=on  Ron_ideal_switch=Rds_on  Vth=Vth  Vgamma=Vdon_diode  Rdon_diode=Rdon_diode  Csnubber=Csnubber  Rsnubber=Rsnubber
  three_phase_inverter_mosfet_based_with_thermal_model : three_phase_inverter_mosfet_based_with_thermal_model/three phase inverter mosfet based with thermal model  mass_heatsink=weigth  specific_heat=cp_al  rth_mosfet_HA=Rth_mosfet_HA  rth_mosfet_JH=dab.Rth_mosfet_JH  Rds_on=dab.Rds_on  Vth=dab.Vth  Eon=dab.Eon  Eoff=dab.Eoff  Voff_sw_loss=dab.Voff_sw_losses  Ion_sw_loss=dab.Ion_sw_losses  Vdon_diode=dab.Vdon_diode  Rdon_diode=dab.Rdon_diode  JunctionTermalMass=dab.JunctionTermalMass  Tambient=Tambient  DThs_init=DThs_init
  udc(+) : PMIOPort  Side=Left
  u : PMIOPort  Port=2  Side=Right
  v : PMIOPort  Port=3  Side=Right
  udc(-) : PMIOPort  Port=4  Side=Left
  w : PMIOPort  Port=5  Side=Right
  tag scope: inverter_1_dab_devices_modA=global
  wires:
  gate_commands/1 -> three_phase_inverter_ideal_switch_based_model/1, three_phase_inverter_mosfet_based_with_thermal_model/1
  three_phase_inverter_mosfet_based_with_thermal_model/1 -> [inverter_1_dab_devices_modA]
  connections:
  u/RConn1 -- three_phase_inverter_ideal_switch_based_model/RConn1 -- three_phase_inverter_mosfet_based_with_thermal_model/RConn1
  v/RConn1 -- three_phase_inverter_ideal_switch_based_model/RConn2 -- three_phase_inverter_mosfet_based_with_thermal_model/RConn2
  udc(-)/RConn1 -- three_phase_inverter_ideal_switch_based_model/LConn2 -- three_phase_inverter_mosfet_based_with_thermal_model/LConn2
  w/RConn1 -- three_phase_inverter_ideal_switch_based_model/RConn3 -- three_phase_inverter_mosfet_based_with_thermal_model/RConn3
  udc(+)/RConn1 -- three_phase_inverter_ideal_switch_based_model/LConn1 -- three_phase_inverter_mosfet_based_with_thermal_model/LConn1

== system sst_three_phase_dab_three_levels_inv/dab_modA/dcdc_with_galvanic_isolation/three_phase_inverter_2/dclink_2 ==
  CFi_dc2 : fl_lib/Electrical/Electrical Elements/Capacitor  c=CFi_dc2 F  r=RCFi_dc2_internal Ohm  g=0 1/Ohm  i_specify=off  i_priority=None  i=0 A  i_nominal_specify=off  i_nominal_value=1  i_nominal_unit=A  v_specify=off  v_priority=None  v=0 V  v_nominal_specify=off  v_nominal_value=1  v_nominal_unit=V  vc_specify=off  vc_priority=High  vc=0 V  vc_nominal_specify=off  vc_nominal_value=1  vc_nominal_unit=V
  Current Sensor2 : fl_lib/Electrical/Electrical Sensors/Current Sensor
  PS-Simulink Converter6 : nesl_utility/PS-Simulink Converter  PhysicalDomain=network_engine_domain  SubClassName=ps_output  LeftPortType=input  RightPortType=output  PseudoPeriodic=off  Frequencies=[]  VectorFormat=1-D array  Unit=A  AffineConversion=on
  ui_measure : Subsystem
  Udc(+) : PMIOPort  Side=Left
  Udc(-) : PMIOPort  Port=2  Side=Left
  udc(+) : PMIOPort  Port=3  Side=Right
  udc(-) : PMIOPort  Port=4  Side=Right
  tag scope: CFi_dc2_current_modA=global
  wires:
  PS-Simulink Converter6/1 -> [CFi_dc2_current_modA]  "CFi_dc2_current_modA"
  connections:
  CFi_dc2/RConn1 -- Current Sensor2/LConn1
  PS-Simulink Converter6/LConn1 -- Current Sensor2/RConn1
  Current Sensor2/RConn2 -- ui_measure/LConn2 -- Udc(-)/RConn1
  CFi_dc2/LConn1 -- ui_measure/LConn1 -- Udc(+)/RConn1
  ui_measure/RConn2 -- udc(-)/RConn1
  ui_measure/RConn1 -- udc(+)/RConn1

== system sst_three_phase_dab_three_levels_inv/dab_modA/dcdc_with_galvanic_isolation/three_phase_inverter_2/three_phase_inverter_2 ==
  gate_commands : Inport
  three_phase_inverter_ideal_switch_based_model : three_phase_inverter_ideal_switch_based_model/three phase inverter ideal switch based model  Commented=on  Ron_ideal_switch=Rds_on  Vth=Vth  Vgamma=Vdon_diode  Rdon_diode=Rdon_diode  Csnubber=Csnubber  Rsnubber=Rsnubber
      link override ideal_switch_3: SourceBlock=three_phase_inverter_ideal_switch_based_model/three_phase_inverter_ideal_switch_based_model/ideal_switch_1
  three_phase_inverter_mosfet_based_with_thermal_model : three_phase_inverter_mosfet_based_with_thermal_model/three phase inverter mosfet based with thermal model  mass_heatsink=weigth  specific_heat=cp_al  rth_mosfet_HA=Rth_mosfet_HA  rth_mosfet_JH=dab.Rth_mosfet_JH  Rds_on=dab.Rds_on  Vth=dab.Vth  Eon=dab.Eon  Eoff=dab.Eoff  Voff_sw_loss=dab.Voff_sw_losses  Ion_sw_loss=dab.Ion_sw_losses  Vdon_diode=dab.Vdon_diode  Rdon_diode=dab.Rdon_diode  JunctionTermalMass=dab.JunctionTermalMass  Tambient=Tambient  DThs_init=DThs_init
  udc(+) : PMIOPort  Side=Right
  u : PMIOPort  Port=2  Side=Left
  v : PMIOPort  Port=3  Side=Left
  udc(-) : PMIOPort  Port=4  Side=Right
  w : PMIOPort  Port=5  Side=Left
  tag scope: inverter_2_dab_devices_modA=global
  wires:
  gate_commands/1 -> three_phase_inverter_ideal_switch_based_model/1, three_phase_inverter_mosfet_based_with_thermal_model/1
  three_phase_inverter_mosfet_based_with_thermal_model/1 -> [inverter_2_dab_devices_modA]
  connections:
  three_phase_inverter_mosfet_based_with_thermal_model/LConn2 -- three_phase_inverter_ideal_switch_based_model/LConn2 -- udc(-)/RConn1
  three_phase_inverter_mosfet_based_with_thermal_model/LConn1 -- udc(+)/RConn1 -- three_phase_inverter_ideal_switch_based_model/LConn1
  three_phase_inverter_mosfet_based_with_thermal_model/RConn1 -- u/RConn1 -- three_phase_inverter_ideal_switch_based_model/RConn1
  three_phase_inverter_mosfet_based_with_thermal_model/RConn3 -- w/RConn1 -- three_phase_inverter_ideal_switch_based_model/RConn3
  three_phase_inverter_mosfet_based_with_thermal_model/RConn2 -- v/RConn1 -- three_phase_inverter_ideal_switch_based_model/RConn2

== system sst_three_phase_dab_three_levels_inv/dab_modB/dab_ctrl/ui_ctrl/dab_ctrl ==
  i_pu_dab_input : Inport
  u_pu_dab_output : Inport  Port=2
  u_pu_dab_output_ref : Inport  Port=3
  Quantizer1 : Quantizer  QuantizationInterval=adc12_quantization
  Quantizer2 : Quantizer  QuantizationInterval=adc12_quantization
  Unit Delay1 : UnitDelay  SampleTime=-1  HasFrameUpgradeWarning=on
  Unit Delay2 : UnitDelay  SampleTime=-1  HasFrameUpgradeWarning=on
  Unit Delay3 : UnitDelay  SampleTime=-1  HasFrameUpgradeWarning=on
  Vout Ctrl : Subsystem
  current control : Subsystem
  discrete-time-low-pass-filter6 : discrete_time_low_pass_filter/discrete-time-low-pass-filter  tau=0.02  ts=ts_dab
  phase_displacement : Outport
  tag scope: i_ctrl_out_dab=scoped, i_in_pu_dab=scoped, u_ctrl_out_dab=scoped, uout_pu_dab=scoped, uout_ref_pu_dab=scoped
  wires:
  Quantizer2/1 -> Unit Delay3/1
  Quantizer1/1 -> Unit Delay2/1
  u_pu_dab_output_ref/1 -> discrete-time-low-pass-filter6/1
  u_pu_dab_output/1 -> Quantizer1/1
  Unit Delay1/1 -> [uout_ref_pu_dab], Vout Ctrl/1(vout_ref)
  Unit Delay2/1 -> Vout Ctrl/2(vout), [uout_pu_dab]
  Unit Delay3/1 -> [i_in_pu_dab], current control/2(iout)
  current control/1(i_ctrl_out) -> [i_ctrl_out_dab], phase_displacement/1
  i_pu_dab_input/1 -> Quantizer2/1
  Vout Ctrl/1(ctrlv_out) -> current control/1(iout_ref), [u_ctrl_out_dab]  "iout_ref"
  discrete-time-low-pass-filter6/1 -> Unit Delay1/1

== system sst_three_phase_dab_three_levels_inv/dab_modB/dab_ctrl/ui_ctrl/scopes ==
  Bus Creator : BusCreator  Inputs=2
  Bus Creator1 : BusCreator  Inputs=2
  dab-tracking : Scope  NumInputPorts=2
      settings: ActiveDisplayYMinimum=-2.3268130293516371  ActiveDisplayYMaximum=3.0115670177424061  DataLoggingVariableName=ScopeData7
  u_ctrl_out_dab/i_ctrl_out_dab : Scope  NumInputPorts=2
      settings: ActiveDisplayYMinimum=-1.2812486231311795  ActiveDisplayYMaximum=1.531237608180616
  wires:
  [uout_pu_dab] -> Bus Creator/2  "uout_pu_dab"
  [u_ctrl_out_dab] -> Bus Creator1/1  "u_ctrl_out_dab"
  [u_ctrl_out_dab] -> u_ctrl_out_dab/i_ctrl_out_dab/1  "u_ctrl_out_dab"
  [uout_ref_pu_dab] -> Bus Creator/1  "uout_ref_pu_dab"
  [i_in_pu_dab] -> Bus Creator1/2  "i_in_pu_dab"
  [i_ctrl_out_dab] -> u_ctrl_out_dab/i_ctrl_out_dab/2  "i_ctrl_out_dab"
  Bus Creator/1 -> dab-tracking/1
  Bus Creator1/1 -> dab-tracking/2

== system sst_three_phase_dab_three_levels_inv/dab_modB/dab_ctrl/ui_ctrl/storage_data ==
  To Workspace1 : ToWorkspace  VariableName=time_ts_dab_modB_sim  SampleTime=-1
      settings: MaxDataPoints=Ns_dab
  To Workspace2 : ToWorkspace  VariableName=i_in_pu_dab_modB_sim  SampleTime=-1
      settings: MaxDataPoints=Ns_dab
  To Workspace3 : ToWorkspace  VariableName=i_in_pu_ref_dab_modB_sim  SampleTime=-1
      settings: MaxDataPoints=Ns_dab
  To Workspace4 : ToWorkspace  VariableName=i_ctrl_out_dab_modB_sim  SampleTime=-1
      settings: MaxDataPoints=Ns_dab
  wires:
  [local_time] -> To Workspace1/1  "local_time"
  [i_in_pu_dab] -> To Workspace2/1  "i_in_pu_dab"
  [i_ctrl_out_dab] -> To Workspace4/1  "i_ctrl_out_dab"
  [u_ctrl_out_dab] -> To Workspace3/1  "u_ctrl_out_dab"

== system sst_three_phase_dab_three_levels_inv/dab_modB/dcdc_with_galvanic_isolation/single_phase_dab_transformer/three_phase_hf_transformer ==
  single_phase_transformer_1 : single_phase_transformer/single_phase_transformer  lm_trafo=lm_trafo  m1=m1  m2=m2  rd1_trafo=rd1_trafo  rd2_trafo=rd2_trafo  ld1_trafo=ld1_trafo  ld2_trafo=ld2_trafo  rfe_trafo=rfe_trafo  length_core=1  mu0=1.256637e-6  mur=10e3
  single_phase_transformer_2 : single_phase_transformer/single_phase_transformer  lm_trafo=lm_trafo  m1=m1  m2=m2  rd1_trafo=rd1_trafo  rd2_trafo=rd2_trafo  ld1_trafo=ld1_trafo  ld2_trafo=ld2_trafo  rfe_trafo=rfe_trafo  length_core=1  mu0=1.256637e-6  mur=10e3
  single_phase_transformer_2: data : Scope
      settings: ActiveDisplayYMinimum=-1744.0416508829171  ActiveDisplayYMaximum=1756.9104494327478  DataLoggingVariableName=ScopeData15
  single_phase_transformer_3 : single_phase_transformer/single_phase_transformer  lm_trafo=lm_trafo  m1=m1  m2=m2  rd1_trafo=rd1_trafo  rd2_trafo=rd2_trafo  ld1_trafo=ld1_trafo  ld2_trafo=ld2_trafo  rfe_trafo=rfe_trafo  length_core=1  mu0=1.256637e-6  mur=10e3
  ua1 : PMIOPort  Side=Left
  ua2 : PMIOPort  Port=2  Side=Right
  ub1 : PMIOPort  Port=3  Side=Left
  ub2 : PMIOPort  Port=4  Side=Right
  uc1 : PMIOPort  Port=5  Side=Left
  uc2 : PMIOPort  Port=6  Side=Right
  un1 : PMIOPort  Port=7  Side=Left
  un2 : PMIOPort  Port=8  Side=Right
  wires:
  single_phase_transformer_2/1 -> single_phase_transformer_2: data/1
  connections:
  single_phase_transformer_1/RConn1 -- ua2/RConn1
  single_phase_transformer_2/RConn1 -- ub2/RConn1
  single_phase_transformer_3/RConn1 -- uc2/RConn1
  single_phase_transformer_3/LConn1 -- uc1/RConn1
  single_phase_transformer_2/LConn1 -- ub1/RConn1
  single_phase_transformer_1/LConn1 -- ua1/RConn1
  single_phase_transformer_3/LConn2 -- single_phase_transformer_1/LConn2 -- single_phase_transformer_2/LConn2 -- un1/RConn1
  single_phase_transformer_3/RConn2 -- single_phase_transformer_1/RConn2 -- single_phase_transformer_2/RConn2 -- un2/RConn1

== system sst_three_phase_dab_three_levels_inv/dab_modB/dcdc_with_galvanic_isolation/single_phase_dab_transformer/threephase_vi_measures_stack ==
  Bus Creator : BusCreator  Inputs=6
  Current Sensor : fl_lib/Electrical/Electrical Sensors/Current Sensor
  Current Sensor1 : fl_lib/Electrical/Electrical Sensors/Current Sensor
  Current Sensor2 : fl_lib/Electrical/Electrical Sensors/Current Sensor
  Gain : Gain  Gain=1/3
  Selector : Selector  InputPortWidth=6  IndexOptions=Index vector (dialog)  Indices=[1 2 3]  OutputSizes=1
  Selector1 : Selector  InputPortWidth=6  IndexOptions=Index vector (dialog)  Indices=[4 5 6]  OutputSizes=1
  Sum : Sum  Inputs=+++
  Voltage Sensor : fl_lib/Electrical/Electrical Sensors/Voltage Sensor
  Voltage Sensor1 : fl_lib/Electrical/Electrical Sensors/Voltage Sensor
  Voltage Sensor2 : fl_lib/Electrical/Electrical Sensors/Voltage Sensor
  ia1 : nesl_utility/PS-Simulink Converter  PhysicalDomain=network_engine_domain  SubClassName=ps_output  LeftPortType=input  RightPortType=output  PseudoPeriodic=off  Frequencies=[]  VectorFormat=1-D array  Unit=A  AffineConversion=off
  ib1 : nesl_utility/PS-Simulink Converter  PhysicalDomain=network_engine_domain  SubClassName=ps_output  LeftPortType=input  RightPortType=output  PseudoPeriodic=off  Frequencies=[]  VectorFormat=1-D array  Unit=A  AffineConversion=off
  ic1 : nesl_utility/PS-Simulink Converter  PhysicalDomain=network_engine_domain  SubClassName=ps_output  LeftPortType=input  RightPortType=output  PseudoPeriodic=off  Frequencies=[]  VectorFormat=1-D array  Unit=A  AffineConversion=off
  ua1 : nesl_utility/PS-Simulink Converter  PhysicalDomain=network_engine_domain  SubClassName=ps_output  LeftPortType=input  RightPortType=output  PseudoPeriodic=off  Frequencies=[]  VectorFormat=1-D array  Unit=V  AffineConversion=off
  ub1 : nesl_utility/PS-Simulink Converter  PhysicalDomain=network_engine_domain  SubClassName=ps_output  LeftPortType=input  RightPortType=output  PseudoPeriodic=off  Frequencies=[]  VectorFormat=1-D array  Unit=V  AffineConversion=off
  uc1 : nesl_utility/PS-Simulink Converter  PhysicalDomain=network_engine_domain  SubClassName=ps_output  LeftPortType=input  RightPortType=output  PseudoPeriodic=off  Frequencies=[]  VectorFormat=1-D array  Unit=V  AffineConversion=off
  Ua : PMIOPort  Side=Left
  ua : PMIOPort  Port=2  Side=Right
  Ub : PMIOPort  Port=3  Side=Left
  ub : PMIOPort  Port=4  Side=Right
  Uc : PMIOPort  Port=5  Side=Left
  uc : PMIOPort  Port=6  Side=Right
  un : PMIOPort  Port=7  Side=Right
  tag scope: i1_dab_transformer_modB=global, u10_dab_transformer_modB=global, u1_dab_transformer_modB=global
  wires:
  Gain/1 -> [u10_dab_transformer_modB]
  Sum/1 -> Gain/1
  Selector1/1 -> [i1_dab_transformer_modB]
  uc1/1 -> Bus Creator/3  "uw1"
  ub1/1 -> Bus Creator/2  "uv1"
  ua1/1 -> Bus Creator/1  "uu1"
  ic1/1 -> Sum/3, Bus Creator/6  "iw1"
  ia1/1 -> Bus Creator/4, Sum/1  "iu1"
  ib1/1 -> Bus Creator/5, Sum/2  "iv1"
  Selector/1 -> [u1_dab_transformer_modB]
  Bus Creator/1 -> Selector1/1, Selector/1  "vi_data"
  connections:
  Current Sensor2/RConn2 -- uc/RConn1
  ic1/LConn1 -- Current Sensor2/RConn1
  ia1/LConn1 -- Current Sensor/RConn1
  ib1/LConn1 -- Current Sensor1/RConn1
  Voltage Sensor2/RConn1 -- uc1/LConn1
  Current Sensor1/RConn2 -- ub/RConn1
  Voltage Sensor/LConn1 -- Ua/RConn1 -- Current Sensor/LConn1
  Current Sensor2/LConn1 -- Uc/RConn1 -- Voltage Sensor2/LConn1
  Voltage Sensor1/RConn1 -- ub1/LConn1
  Current Sensor/RConn2 -- ua/RConn1
  Voltage Sensor/RConn1 -- ua1/LConn1
  Voltage Sensor1/RConn2 -- Voltage Sensor2/RConn2 -- un/RConn1 -- Voltage Sensor/RConn2
  Voltage Sensor1/LConn1 -- Ub/RConn1 -- Current Sensor1/LConn1

== system sst_three_phase_dab_three_levels_inv/dab_modB/dcdc_with_galvanic_isolation/single_phase_dab_transformer/threephase_vi_measures_stack1 ==
  Bus Creator : BusCreator  Inputs=6
  Current Sensor : fl_lib/Electrical/Electrical Sensors/Current Sensor
  Current Sensor1 : fl_lib/Electrical/Electrical Sensors/Current Sensor
  Current Sensor2 : fl_lib/Electrical/Electrical Sensors/Current Sensor
  Gain : Gain  Gain=1/3
  Selector : Selector  InputPortWidth=6  IndexOptions=Index vector (dialog)  Indices=[1 2 3]  OutputSizes=1
  Selector1 : Selector  InputPortWidth=6  IndexOptions=Index vector (dialog)  Indices=[4 5 6]  OutputSizes=1
  Sum : Sum  Inputs=+++
  Voltage Sensor : fl_lib/Electrical/Electrical Sensors/Voltage Sensor
  Voltage Sensor1 : fl_lib/Electrical/Electrical Sensors/Voltage Sensor
  Voltage Sensor2 : fl_lib/Electrical/Electrical Sensors/Voltage Sensor
  iu : nesl_utility/PS-Simulink Converter  PhysicalDomain=network_engine_domain  SubClassName=ps_output  LeftPortType=input  RightPortType=output  PseudoPeriodic=off  Frequencies=[]  VectorFormat=1-D array  Unit=A  AffineConversion=off
  iv : nesl_utility/PS-Simulink Converter  PhysicalDomain=network_engine_domain  SubClassName=ps_output  LeftPortType=input  RightPortType=output  PseudoPeriodic=off  Frequencies=[]  VectorFormat=1-D array  Unit=A  AffineConversion=off
  iw : nesl_utility/PS-Simulink Converter  PhysicalDomain=network_engine_domain  SubClassName=ps_output  LeftPortType=input  RightPortType=output  PseudoPeriodic=off  Frequencies=[]  VectorFormat=1-D array  Unit=A  AffineConversion=off
  uu : nesl_utility/PS-Simulink Converter  PhysicalDomain=network_engine_domain  SubClassName=ps_output  LeftPortType=input  RightPortType=output  PseudoPeriodic=off  Frequencies=[]  VectorFormat=1-D array  Unit=V  AffineConversion=off
  uv : nesl_utility/PS-Simulink Converter  PhysicalDomain=network_engine_domain  SubClassName=ps_output  LeftPortType=input  RightPortType=output  PseudoPeriodic=off  Frequencies=[]  VectorFormat=1-D array  Unit=V  AffineConversion=off
  uw : nesl_utility/PS-Simulink Converter  PhysicalDomain=network_engine_domain  SubClassName=ps_output  LeftPortType=input  RightPortType=output  PseudoPeriodic=off  Frequencies=[]  VectorFormat=1-D array  Unit=V  AffineConversion=off
  Ua : PMIOPort  Side=Left
  ua : PMIOPort  Port=2  Side=Right
  Ub : PMIOPort  Port=3  Side=Left
  ub : PMIOPort  Port=4  Side=Right
  Uc : PMIOPort  Port=5  Side=Left
  uc : PMIOPort  Port=6  Side=Right
  Un : PMIOPort  Port=7  Side=Left
  tag scope: i2_dab0_transformer_modB=global, i2_dab_transformer_modB=global, u2_dab_transformer_modB=global
  wires:
  Bus Creator/1 -> Selector/1, Selector1/1  "vi_data"
  Selector/1 -> [u2_dab_transformer_modB]
  iv/1 -> Sum/2, Bus Creator/5  "iv2"
  iu/1 -> Sum/1, Bus Creator/4  "iu2"
  iw/1 -> Sum/3, Bus Creator/6  "iw2"
  uv/1 -> Bus Creator/2  "uv2"
  uw/1 -> Bus Creator/3  "uw2"
  Selector1/1 -> [i2_dab_transformer_modB]
  Sum/1 -> Gain/1
  Gain/1 -> [i2_dab0_transformer_modB]
  uu/1 -> Bus Creator/1  "uu2"
  connections:
  Current Sensor1/LConn1 -- Ub/RConn1 -- Voltage Sensor1/LConn1
  Voltage Sensor/RConn2 -- Voltage Sensor2/RConn2 -- Un/RConn1 -- Voltage Sensor1/RConn2
  Voltage Sensor/RConn1 -- uu/LConn1
  Current Sensor/RConn2 -- ua/RConn1
  Voltage Sensor1/RConn1 -- uv/LConn1
  Voltage Sensor2/LConn1 -- Uc/RConn1 -- Current Sensor2/LConn1
  Current Sensor/LConn1 -- Ua/RConn1 -- Voltage Sensor/LConn1
  Current Sensor1/RConn2 -- ub/RConn1
  Voltage Sensor2/RConn1 -- uw/LConn1
  iv/LConn1 -- Current Sensor1/RConn1
  iu/LConn1 -- Current Sensor/RConn1
  iw/LConn1 -- Current Sensor2/RConn1
  Current Sensor2/RConn2 -- uc/RConn1

== system sst_three_phase_dab_three_levels_inv/dab_modB/dcdc_with_galvanic_isolation/three_phase_inverter_1/dclink_1 ==
  CFi_dc1 : fl_lib/Electrical/Electrical Elements/Capacitor  c=CFi_dc1 F  r=RCFi_dc1_internal Ohm  g=0 1/Ohm  i_specify=off  i_priority=None  i=0 A  i_nominal_specify=off  i_nominal_value=1  i_nominal_unit=A  v_specify=off  v_priority=None  v=0 V  v_nominal_specify=off  v_nominal_value=1  v_nominal_unit=V  vc_specify=off  vc_priority=High  vc=0 V  vc_nominal_specify=off  vc_nominal_value=1  vc_nominal_unit=V
  Current Sensor : fl_lib/Electrical/Electrical Sensors/Current Sensor
  PS-Simulink Converter4 : nesl_utility/PS-Simulink Converter  PhysicalDomain=network_engine_domain  SubClassName=ps_output  LeftPortType=input  RightPortType=output  PseudoPeriodic=off  Frequencies=[]  VectorFormat=1-D array  Unit=V  AffineConversion=on
  Voltage Sensor : fl_lib/Electrical/Electrical Sensors/Voltage Sensor
  udc(+) : PMIOPort  Side=Left
  Udc(+) : PMIOPort  Port=2  Side=Right
  udc(-) : PMIOPort  Port=3  Side=Left
  Udc(-) : PMIOPort  Port=4  Side=Right
  tag scope: dab_voltage_input_modB=global
  wires:
  PS-Simulink Converter4/1 -> [dab_voltage_input_modB]  "dab_voltage_input_modA"
  connections:
  Voltage Sensor/LConn1 -- udc(+)/RConn1 -- Udc(+)/RConn1 -- CFi_dc1/LConn1
  udc(-)/RConn1 -- Udc(-)/RConn1 -- Current Sensor/RConn2 -- Voltage Sensor/RConn2
  Current Sensor/LConn1 -- CFi_dc1/RConn1
  PS-Simulink Converter4/LConn1 -- Voltage Sensor/RConn1

== system sst_three_phase_dab_three_levels_inv/dab_modB/dcdc_with_galvanic_isolation/three_phase_inverter_1/three_phase_inverter_1 ==
  gate_commands : Inport
  three_phase_inverter_ideal_switch_based_model : three_phase_inverter_ideal_switch_based_model/three phase inverter ideal switch based model  Ron_ideal_switch=Rds_on  Vth=Vth  Vgamma=Vdon_diode  Rdon_diode=Rdon_diode  Csnubber=Csnubber  Rsnubber=Rsnubber
  three_phase_inverter_mosfet_based_with_thermal_model : three_phase_inverter_mosfet_based_with_thermal_model/three phase inverter mosfet based with thermal model  Commented=on  mass_heatsink=0.2  specific_heat=cp_al  rth_mosfet_HA=Rth_mosfet_HA  rth_mosfet_JH=Rth_mosfet_JH  Rds_on=Rds_on  Vth=Vth  Eon=Eon  Eoff=Eoff  Voff_sw_loss=Voff_sw_losses  Ion_sw_loss=Ion_sw_losses  Vdon_diode=Vdon_diode  Rdon_diode=Rdon_diode  JunctionTermalMass=JunctionTermalMass  Tambient=Tambient  DThs_init=DThs_init
  udc(+) : PMIOPort  Side=Left
  u : PMIOPort  Port=2  Side=Right
  v : PMIOPort  Port=3  Side=Right
  udc(-) : PMIOPort  Port=4  Side=Left
  w : PMIOPort  Port=5  Side=Right
  tag scope: inverter_1_dab_devices_modB=global
  wires:
  three_phase_inverter_mosfet_based_with_thermal_model/1 -> [inverter_1_dab_devices_modB]
  gate_commands/1 -> three_phase_inverter_mosfet_based_with_thermal_model/1, three_phase_inverter_ideal_switch_based_model/1
  connections:
  three_phase_inverter_mosfet_based_with_thermal_model/LConn1 -- three_phase_inverter_ideal_switch_based_model/LConn1 -- udc(+)/RConn1
  three_phase_inverter_mosfet_based_with_thermal_model/RConn3 -- three_phase_inverter_ideal_switch_based_model/RConn3 -- w/RConn1
  three_phase_inverter_mosfet_based_with_thermal_model/LConn2 -- three_phase_inverter_ideal_switch_based_model/LConn2 -- udc(-)/RConn1
  three_phase_inverter_mosfet_based_with_thermal_model/RConn2 -- three_phase_inverter_ideal_switch_based_model/RConn2 -- v/RConn1
  three_phase_inverter_mosfet_based_with_thermal_model/RConn1 -- three_phase_inverter_ideal_switch_based_model/RConn1 -- u/RConn1
